simulink model "REPFF_sim"  (R2022b)
settings: Solver=FixedStepAuto  StartTime=0.0  StopTime=time_final  RelTol=1e-3
values from neighbouring files (symbols this model uses):
  Fzpet_den = F.Denominator{1}    [REPFF.m]
  Fzpet_num = F.Numerator{1}    [REPFF.m]
  K_aug = [K_SF,K_int]    [control_design.m]
  NF = NF + Nw    (= 27)    [REPFF.m]
  signal_num = 2    [REPFF.m]    (also in REPFF_test.m)
  Stepsize = 0.4    [REPFF.m]    (also in REPFF_test.m; system_id_CLSOFCI.m)
  Tcomp = 0.0005*Ts*14    (= 7e-06)    [REPFF.m]
  time_step = 10    [REPFF.m]    (also in REPFF_test.m; system_id_CLSOFCI.m)
  Ts = 0.001    [REPFF.m]    (also in REPFF_test.m; control_design.m; system_id_CLSOFCI.m)
  Tss = 1/10000    (= 0.0001)    [REPFF.m]
  unit_period = 1    [REPFF.m]    (also in REPFF_test.m)
  W_coe = W.Numerator{1}/W.Denominator{1}(Nw+1)    [REPFF.m]
undefined symbols (not defined in the file or in its folder): A_d, Ad, b, B_d, Bd, C_d, L, L_Pred, N, R
libraries: simulink x1
settings Model: Creator=Alex Zhen  LastModifiedBy=Alex Zhen
settings SolverCC: ZeroCrossControl=DisableAll  ZeroCrossAlgorithm=Adaptive
settings DebuggingCC: IgnoredZcDiagnostic=none

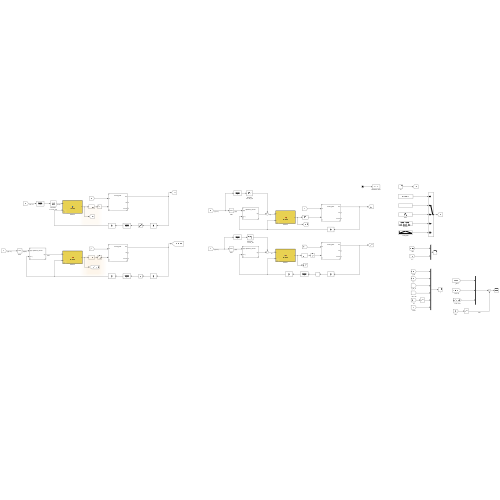
[thumbnail: Simulink's stored preview of the top-level diagram]
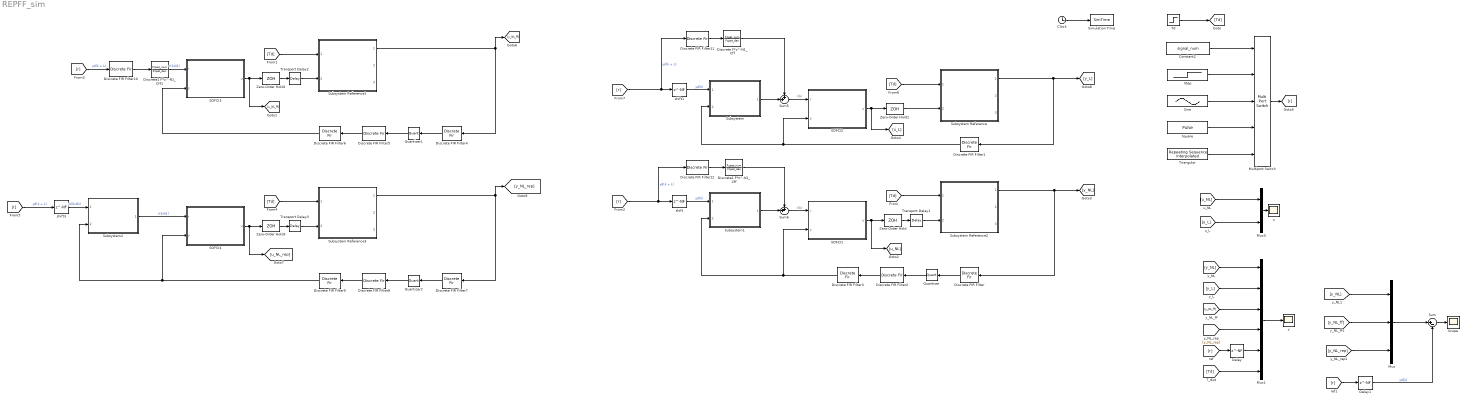
== system REPFF_sim ==
  Clock : Clock
  Constant2 : Constant  Value=signal_num
  Delay : Delay  DelayLength=NF
  Delay1 : Delay  DelayLength=NF
  Discrete F*z^-N1_Cff : DiscreteTransferFcn  Numerator=Fzpet_num  Denominator=Fzpet_den  SampleTime=Ts
  Discrete FIR Filter : DiscreteFir  Coefficients=[1]  SampleTime=Tss
  Discrete FIR Filter{1,3,6,9} (4 alike) : DiscreteFir  Coefficients=[1]  SampleTime=Ts
  Discrete FIR Filter10 : DiscreteFir  Coefficients=W_coe
  Discrete FIR Filter11 : DiscreteFir  Coefficients=W_coe
  Discrete FIR Filter12 : DiscreteFir  Coefficients=W_coe
  Discrete FIR Filter2 : DiscreteFir  Coefficients=[0.25 0.25 0.25 0.25]
  Discrete FIR Filter4 : DiscreteFir  Coefficients=[1]  SampleTime=Tss
  Discrete FIR Filter5 : DiscreteFir  Coefficients=[0.25 0.25 0.25 0.25]
  Discrete FIR Filter7 : DiscreteFir  Coefficients=[1]  SampleTime=Tss
  Discrete FIR Filter8 : DiscreteFir  Coefficients=[0.25 0.25 0.25 0.25]
  Discrete1 F*z^-N1_Cff : DiscreteTransferFcn  Numerator=Fzpet_num  Denominator=Fzpet_den  SampleTime=Ts
  Discrete1 F*z^-N1_Cff1 : DiscreteTransferFcn  Numerator=Fzpet_num  Denominator=Fzpet_den  SampleTime=Ts
  Multiport Switch : MultiPortSwitch  Inputs=4  SaturateOnIntegerOverflow=off  InputSameDT=off
  Mux : Mux  Inputs=3
  Mux1 : Mux  Inputs=6
  Mux3 : Mux  Inputs=2
  Quantizer : Quantizer  QuantizationInterval=encoder_resolution
  Quantizer1 : Quantizer  QuantizationInterval=encoder_resolution
  Quantizer2 : Quantizer  QuantizationInterval=encoder_resolution
  SOFCI1 : MATLAB Function  TreatAsAtomicUnit=on  mask{A=A_d, B=B_d, C=C_d, K=K_aug, L=L_Pred, N=N, Ad=Ad, Bd=Bd, linear_nonlinear=Nonlinear}
      mask prompts: linear_nonlinear "Linear/Nonlinear"
  SOFCI2 : MATLAB Function  TreatAsAtomicUnit=on  mask{A=A_d, B=B_d, C=C_d, K=K_aug, L=L_Pred, N=N, Ad=Ad, Bd=Bd, linear_nonlinear=Linear}
      mask prompts: linear_nonlinear "Linear/Nonlinear"
  SOFCI3 : MATLAB Function  TreatAsAtomicUnit=on  mask{A=A_d, B=B_d, C=C_d, K=K_aug, L=L_Pred, N=N, Ad=Ad, Bd=Bd, linear_nonlinear=Nonlinear}
      mask prompts: linear_nonlinear "Linear/Nonlinear"
  SOFCI4 : MATLAB Function  TreatAsAtomicUnit=on  mask{A=A_d, B=B_d, C=C_d, K=K_aug, L=L_Pred, N=N, Ad=Ad, Bd=Bd, linear_nonlinear=Nonlinear}
      mask prompts: linear_nonlinear "Linear/Nonlinear"
  Scope : Scope
  Simulation Time : ToWorkspace  VariableName=SimTime  SampleTime=-1
  Sine : Sin  Amplitude=Stepsize/2  Bias=Stepsize/2  Frequency=2*pi/(1/unit_period)  SampleTime=Ts
  Square : DiscretePulseGenerator  Amplitude=Stepsize  Period=1/Ts  PulseWidth=1/Ts/2  SampleTime=Ts
  Step : Step  Time=time_step  After=Stepsize  SampleTime=Ts
  Subsystem : Subsystem  ReferencedSubsystem=repetitive_control  Np=Np  N1=N1  N2=N2  Fzpet_num=Fzpet_num  Fzpet_den=Fzpet_den  Q_coe=Q_coe  Qzpet_num=0  Qzpet_den=0
  Subsystem Reference : Subsystem  ReferencedSubsystem=virtual_plant  L=L  K_m=K_m  J_pend=J_pend  b=b  V_s=V_s  R=R  K_pend=K_pend  K_sin=K_sin  K_g=K_g  V_table=V_table  DC_table=DC_table  friction_static=friction_static  friction_viscous=friction_viscous  friction_aero=friction_aero  linear_mode=Linear
  Subsystem Reference1 : Subsystem  ReferencedSubsystem=virtual_plant  L=L  K_m=K_m  J_pend=J_pend  b=b  V_s=V_s  R=R  K_pend=K_pend  K_sin=K_sin  K_g=K_g  V_table=V_table  DC_table=DC_table  friction_static=friction_static  friction_viscous=friction_viscous  friction_aero=friction_aero  linear_mode=Nonlinear
  Subsystem Reference2 : Subsystem  ReferencedSubsystem=virtual_plant  L=L  K_m=K_m  J_pend=J_pend  b=b  V_s=V_s  R=R  K_pend=K_pend  K_sin=K_sin  K_g=K_g  V_table=V_table  DC_table=DC_table  friction_static=friction_static  friction_viscous=friction_viscous  friction_aero=friction_aero  linear_mode=Nonlinear
  Subsystem Reference3 : Subsystem  ReferencedSubsystem=virtual_plant  L=L  K_m=K_m  J_pend=J_pend  b=b  V_s=V_s  R=R  K_pend=K_pend  K_sin=K_sin  K_g=K_g  V_table=V_table  DC_table=DC_table  friction_static=friction_static  friction_viscous=friction_viscous  friction_aero=friction_aero  linear_mode=Nonlinear
  Subsystem1 : Subsystem  ReferencedSubsystem=repetitive_control  Np=Np  N1=N1  N2=N2  Fzpet_num=Fzpet_num  Fzpet_den=Fzpet_den  Q_coe=Q_coe  Qzpet_num=0  Qzpet_den=0
  Subsystem2 : Subsystem  ReferencedSubsystem=repetitive_control  Np=Np  N1=N1  N2=N2  Fzpet_num=Fzpet_num  Fzpet_den=Fzpet_den  Q_coe=Q_coe  Qzpet_num=0  Qzpet_den=0
  Sum : Sum  Inputs=|+-
  Sum5 : Sum  Inputs=++|
  Sum6 : Sum  Inputs=++|
  Td : Step  Time=5  After=0  SampleTime=0
  Transport Delay1 : TransportDelay  DelayTime=Tcomp  BufferSize=4096  PadeOrder=2
  Transport Delay2 : TransportDelay  DelayTime=Tcomp  BufferSize=4096  PadeOrder=2
  Transport Delay3 : TransportDelay  DelayTime=Tcomp  BufferSize=4096  PadeOrder=2
  Triangular : simulink/Sources/Repeating Sequence Interpolated  OutValues=[0 Stepsize 0]  TimeValues=[0 unit_period/2 unit_period]  LookUpMeth=Interpolation-Use End Values  tsamp=Ts  OutMin=[]  OutMax=[]  OutDataTypeStr=double  OutputDataTypeScalingMode=double  OutDataType=fixdt(0,8)  OutScaling=2^-10
  Zero-Order Hold{,1..3} (4 alike) : ZeroOrderHold  SampleTime=Ts
  shift : Delay  DelayLength=NF
  shift1 : Delay  DelayLength=NF
  shift3 : Delay  DelayLength=NF
  u : Scope
  y : Scope
  wires:
  Subsystem Reference2/1 -> [y_NL], Discrete FIR Filter/1
  Transport Delay1/1 -> Subsystem Reference2/2
  [Td] -> Subsystem Reference/1
  Discrete FIR Filter/1 -> Quantizer/1
  Zero-Order Hold/1 -> Transport Delay1/1
  Subsystem Reference/1 -> [y_L], Discrete FIR Filter1/1
  Quantizer/1 -> Discrete FIR Filter2/1
  Discrete FIR Filter2/1 -> Discrete FIR Filter3/1
  Td/1 -> [Td]
  Clock/1 -> Simulation Time/1
  Zero-Order Hold1/1 -> Subsystem Reference/2
  [Td] -> Subsystem Reference2/1
  SOFCI1/1(u) -> [u_NL], Zero-Order Hold/1
  Mux3/1 -> u/1
  [y_L] -> Mux1/2
  [y_NL] -> Mux1/1
  Mux1/1 -> y/1
  [u_L] -> Mux3/2
  [u_NL] -> Mux3/1
  [Td] -> Mux1/6
  Discrete FIR Filter3/1 -> Subsystem1/2, SOFCI1/2(y)
  [r] -> Delay/1
  [r] -> shift/1, Discrete FIR Filter12/1  "yd(k + L)"
  Discrete F*z^-N1_Cff/1 -> Sum5/1
  Sum6/1 -> SOFCI1/1(r)  "r(k)"
  Discrete1 F*z^-N1_Cff/1 -> Sum6/1
  SOFCI2/1(u) -> [u_L], Zero-Order Hold1/1
  Discrete FIR Filter1/1 -> Subsystem/2, SOFCI2/2(y)
  Subsystem/1 -> Sum5/2
  Sum5/1 -> SOFCI2/1(r)  "r(k)"
  [r] -> Discrete FIR Filter11/1, shift1/1  "yd(k + L)"
  shift1/1 -> Subsystem/1  "yd(k)"
  Subsystem1/1 -> Sum6/2
  shift/1 -> Subsystem1/1  "yd(k)"
  Constant2/1 -> Multiport Switch/1
  Sine/1 -> Multiport Switch/3
  Step/1 -> Multiport Switch/2
  Square/1 -> Multiport Switch/4
  Triangular/1 -> Multiport Switch/5
  Multiport Switch/1 -> [r]
  SOFCI3/1(u) -> [u_NL_ff], Zero-Order Hold2/1
  Quantizer1/1 -> Discrete FIR Filter5/1
  [Td] -> Subsystem Reference1/1
  [r] -> Discrete FIR Filter10/1  "yd(k + L)"
  Zero-Order Hold2/1 -> Transport Delay2/1
  Discrete1 F*z^-N1_Cff1/1 -> SOFCI3/1(r)  "r(k-N1)"
  Discrete FIR Filter6/1 -> SOFCI3/2(y)
  Subsystem Reference1/1 -> Discrete FIR Filter4/1, [y_NL_ff]
  Discrete FIR Filter5/1 -> Discrete FIR Filter6/1
  Transport Delay2/1 -> Subsystem Reference1/2
  Discrete FIR Filter4/1 -> Quantizer1/1
  shift3/1 -> Subsystem2/1  "yd(k-N1)"
  SOFCI4/1(u) -> [u_NL_rep], Zero-Order Hold3/1
  Quantizer2/1 -> Discrete FIR Filter8/1
  [Td] -> Subsystem Reference3/1
  [r] -> shift3/1  "yd(k + L)"
  Zero-Order Hold3/1 -> Transport Delay3/1
  Discrete FIR Filter9/1 -> Subsystem2/2, SOFCI4/2(y)
  Subsystem Reference3/1 -> Discrete FIR Filter7/1, [y_NL_rep]
  Discrete FIR Filter8/1 -> Discrete FIR Filter9/1
  Transport Delay3/1 -> Subsystem Reference3/2
  Discrete FIR Filter7/1 -> Quantizer2/1
  Subsystem2/1 -> SOFCI4/1(r)  "r(k-N1)"
  [y_NL_rep] -> Mux/3
  [y_NL] -> Mux/1
  [y_NL_ff] -> Mux/2
  Mux/1 -> Sum/1
  [r] -> Delay1/1
  Delay1/1 -> Sum/2  "yd[k]"
  Sum/1 -> Scope/1
  Discrete FIR Filter10/1 -> Discrete1 F*z^-N1_Cff1/1
  [y_NL_ff] -> Mux1/3
  Discrete FIR Filter11/1 -> Discrete F*z^-N1_Cff/1
  Discrete FIR Filter12/1 -> Discrete1 F*z^-N1_Cff/1
  [y_NL_rep] -> Mux1/4
  Delay/1 -> Mux1/5

== matlab function REPFF_sim/SOFCI1 ==
  data: r input; u output; y input; A parameter; B parameter; C parameter; K parameter; L parameter; N parameter; Ad parameter; Bd parameter; linear_nonlinear parameter
function u = controller(r, y, A, B, C, K, L, N, Ad, Bd, linear_nonlinear)

persistent xhat xint;  %memory for the state

if isempty(xhat)  %local variable initialization
    n=size(L,1);
    xhat=zeros(n,1); 
    m = size(K,2) - n;
    xint=zeros(m,1);  
end

xaug=[xhat; xint]; %Augmented state include the state for the integrator

u_unsat = -K*xaug + N*r; %Control computation with integral action

if linear_nonlinear == 1
    u = u_unsat;
else
    u = sign(u_unsat)*min(1,abs(u_unsat));
end
%Update the next state next
xhat = (A-L*C)*xhat + B*u + L*y;
xint = Ad*xint + Bd*(y - r);

== matlab function REPFF_sim/SOFCI2 ==
  data: r input; u output; y input; A parameter; B parameter; C parameter; K parameter; L parameter; N parameter; Ad parameter; Bd parameter; linear_nonlinear parameter
function u = controller(r, y, A, B, C, K, L, N, Ad, Bd, linear_nonlinear)

persistent xhat xint;  %memory for the state

if isempty(xhat)  %local variable initialization
    n=size(L,1);
    xhat=zeros(n,1); 
    m = size(K,2) - n;
    xint=zeros(m,1);  
end

xaug=[xhat; xint]; %Augmented state include the state for the integrator

u_unsat = -K*xaug + N*r; %Control computation with integral action

if linear_nonlinear == 1
    u = u_unsat;
else
    u = sign(u_unsat)*min(1,abs(u_unsat));
end
%Update the next state next
xhat = (A-L*C)*xhat + B*u + L*y;
xint = Ad*xint + Bd*(y - r);

== matlab function REPFF_sim/SOFCI3 ==
  data: r input; u output; y input; A parameter; B parameter; C parameter; K parameter; L parameter; N parameter; Ad parameter; Bd parameter; linear_nonlinear parameter
function u = controller(r, y, A, B, C, K, L, N, Ad, Bd, linear_nonlinear)

persistent xhat xint;  %memory for the state

if isempty(xhat)  %local variable initialization
    n=size(L,1);
    xhat=zeros(n,1); 
    m = size(K,2) - n;
    xint=zeros(m,1);  
end

xaug=[xhat; xint]; %Augmented state include the state for the integrator

u_unsat = -K*xaug + N*r; %Control computation with integral action

if linear_nonlinear == 1
    u = u_unsat;
else
    u = sign(u_unsat)*min(1,abs(u_unsat));
end
%Update the next state next
xhat = (A-L*C)*xhat + B*u + L*y;
xint = Ad*xint + Bd*(y - r);

== matlab function REPFF_sim/SOFCI4 ==
  data: r input; u output; y input; A parameter; B parameter; C parameter; K parameter; L parameter; N parameter; Ad parameter; Bd parameter; linear_nonlinear parameter
function u = controller(r, y, A, B, C, K, L, N, Ad, Bd, linear_nonlinear)

persistent xhat xint;  %memory for the state

if isempty(xhat)  %local variable initialization
    n=size(L,1);
    xhat=zeros(n,1); 
    m = size(K,2) - n;
    xint=zeros(m,1);  
end

xaug=[xhat; xint]; %Augmented state include the state for the integrator

u_unsat = -K*xaug + N*r; %Control computation with integral action

if linear_nonlinear == 1
    u = u_unsat;
else
    u = sign(u_unsat)*min(1,abs(u_unsat));
end
%Update the next state next
xhat = (A-L*C)*xhat + B*u + L*y;
xint = Ad*xint + Bd*(y - r);
